simulink model "plant_no_lineal"  (R2020a)
settings: Solver=VariableStepAuto  StartTime=0.0  StopTime=5  RelTol=1e-3
settings Model: Creator=estra  LastModifiedBy=User

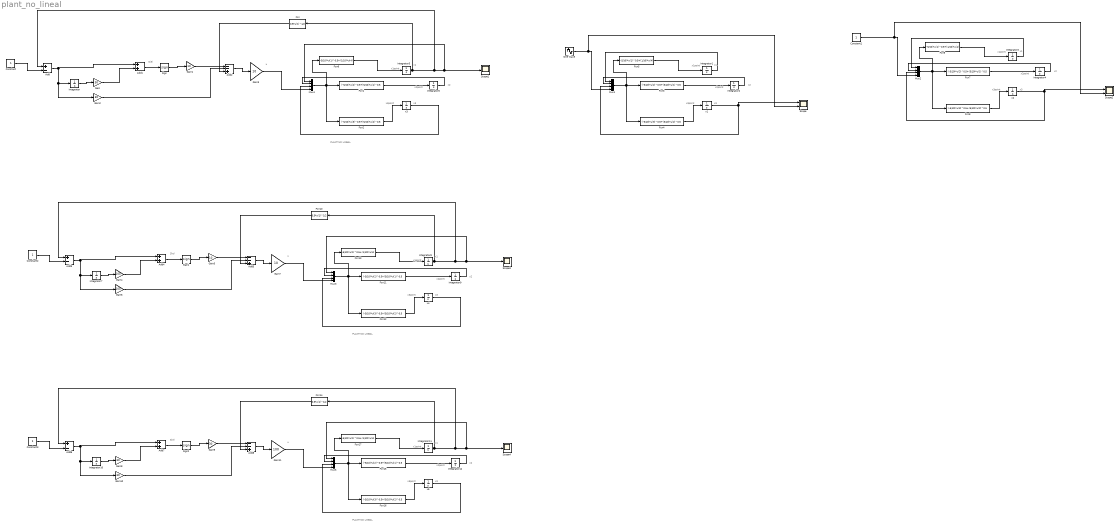
== system plant_no_lineal ==
  note: PLANT NO LINEAL
  note: S(e)
  note: x1
  note: x3
  note: x2
  note: x1point
  note: x2point
  note: x3point
  note: x3point
  note: x1point
  note: x1
  note: x2point
  note: x3
  note: x2
  note: u
  note: x3point
  note: x2point
  note: x1
  note: x3
  note: x1point
  note: x2
  note: x1
  note: PLANT NO LINEAL
  note: x1point
  note: x2point
  note: x3point
  note: x2
  note: x3
  note: S(e)
  note: u
  note: x1
  note: PLANT NO LINEAL
  note: x1point
  note: x2point
  note: x3point
  note: x2
  note: x3
  note: S(e)
  note: u
  Add : Sum  Inputs=+-
  Add1 : Sum
  Add2 : Sum  Inputs=--+
  Add3 : Sum  Inputs=+-
  Add4 : Sum
  Add5 : Sum  Inputs=--+
  Add6 : Sum  Inputs=+-
  Add7 : Sum
  Add8 : Sum  Inputs=--+
  Constant{,1..3} (4 alike) : Constant
  Fcn : Fcn  Expr=0.5*u(1)^1/2
  Fcn{1,3,7,11,15} (5 alike) : Fcn  Expr=(-5/10)*u(2)^0.5+(5/10)*u(1)^0.5
  Fcn10 : Fcn  Expr=0.5*u(1)^1/2
  Fcn{2,4,8,12,16} (5 alike) : Fcn  Expr=(-5/10)*u(3)^0.5+(5/10)*u(2)^0.5
  Fcn{5..6,9,13,17} (5 alike) : Fcn  Expr=(-5/10)*u(1)^0.5+(1/10)*u(4)
  Fcn14 : Fcn  Expr=0.5*u(1)^1/2
  Gain{,2,8..10} (5 alike) : Gain  Gain=30
  Gain{1,3,5,7} (4 alike) : Gain  Gain=10
  Gain11 : Gain  Gain=100
  Gain4 : Gain  Gain=100
  Gain6 : Gain  Gain=100
  Integrator{,1..12} (13 alike) : Integrator
  Mux{1..5} (5 alike) : Mux
  Scope : Scope  NumInputPorts=2
  Scope1 : Scope
  Scope2 : Scope  NumInputPorts=2
  Scope3 : Scope
  Scope4 : Scope
  Sign : Signum  ZeroCross=off
  Sign1 : Signum  ZeroCross=off
  Sign2 : Signum  ZeroCross=off
  Sine Wave : Sin  SampleTime=0
  x{1..5} (5 alike) : Integrator
  wires:
  Fcn6/1 -> Integrator5/1
  Gain3/1 -> Mux4/4
  Fcn1/1 -> Integrator6/1
  Fcn2/1 -> x3/1
  x3/1 -> Mux4/3
  Mux4/1 -> Fcn6/1, Fcn2/1, Fcn1/1
  Integrator6/1 -> Mux4/2
  Mux1/1 -> Fcn5/1, Fcn4/1, Fcn3/1
  Integrator1/1 -> Mux1/1
  x1/1 -> Mux1/3, Scope/1
  Fcn4/1 -> x1/1
  Integrator2/1 -> Mux1/2
  Fcn3/1 -> Integrator2/1
  Fcn5/1 -> Integrator1/1
  Sine Wave/1 -> Scope/2, Mux1/4
  Add/1 -> Add1/1, Gain2/1, Integrator/1
  Integrator/1 -> Gain/1
  Gain/1 -> Add1/2
  Add1/1 -> Sign/1
  Sign/1 -> Gain1/1
  Gain1/1 -> Add2/1
  Gain2/1 -> Add2/2
  Fcn/1 -> Add2/3
  Add2/1 -> Gain3/1
  Constant/1 -> Add/2
  Integrator5/1 -> Fcn/1, Add/1, Mux4/1, Scope1/1
  Constant1/1 -> Scope2/2, Mux2/4
  Fcn8/1 -> x2/1
  Fcn7/1 -> Integrator4/1
  Integrator4/1 -> Mux2/2
  Fcn9/1 -> Integrator3/1
  Mux2/1 -> Fcn9/1, Fcn8/1, Fcn7/1
  x2/1 -> Mux2/3, Scope2/1
  Integrator3/1 -> Mux2/1
  Integrator8/1 -> Fcn10/1, Add3/1, Mux3/1, Scope3/1
  Gain5/1 -> Add5/1
  Add5/1 -> Gain7/1
  Fcn13/1 -> Integrator8/1
  Constant2/1 -> Add3/2
  Fcn10/1 -> Add5/3
  Gain6/1 -> Add5/2
  Mux3/1 -> Fcn13/1, Fcn12/1, Fcn11/1
  Integrator7/1 -> Gain4/1
  Fcn11/1 -> Integrator9/1
  Add4/1 -> Sign1/1
  Gain4/1 -> Add4/2
  Integrator9/1 -> Mux3/2
  Sign1/1 -> Gain5/1
  Add3/1 -> Add4/1, Gain6/1, Integrator7/1
  Gain7/1 -> Mux3/4
  Fcn12/1 -> x4/1
  x4/1 -> Mux3/3
  Integrator11/1 -> Fcn14/1, Add6/1, Mux5/1, Scope4/1
  Gain9/1 -> Add8/1
  Add8/1 -> Gain11/1
  Fcn17/1 -> Integrator11/1
  Constant3/1 -> Add6/2
  Fcn14/1 -> Add8/3
  Gain10/1 -> Add8/2
  Mux5/1 -> Fcn17/1, Fcn16/1, Fcn15/1
  Integrator10/1 -> Gain8/1
  Fcn15/1 -> Integrator12/1
  Add7/1 -> Sign2/1
  Gain8/1 -> Add7/2
  Integrator12/1 -> Mux5/2
  Sign2/1 -> Gain9/1
  Add6/1 -> Add7/1, Gain10/1, Integrator10/1
  Gain11/1 -> Mux5/4
  Fcn16/1 -> x5/1
  x5/1 -> Mux5/3
